simulink model "lab3sl"  (R2020b)
settings: Solver=VariableStepAuto  StartTime=0.0  StopTime=10.0  RelTol=1e-3
values from neighbouring files (symbols this model uses):
  a = t^3 * sin(2*t + pi)    [Laplace.m]    (also in lab3_config1 (1).m = 100)
  am = 1.71    [lab3_config1 (1).m]
  K = dcgain(num2,denum2)    [Lab2.m]    (also in Lab_4.m = 2.43; lab3_config1 (1).m = 22.985)
  K1 = 100    [lab3_config1 (1).m]
  Kg = 0.1    [lab3_config1 (1).m]
  Km = 2.083    [lab3_config1 (1).m]
  Kpot = 0.318    [lab3_config1 (1).m]
libraries: pid_lib x1
settings Model: Creator=mluser  LastModifiedBy=mluser

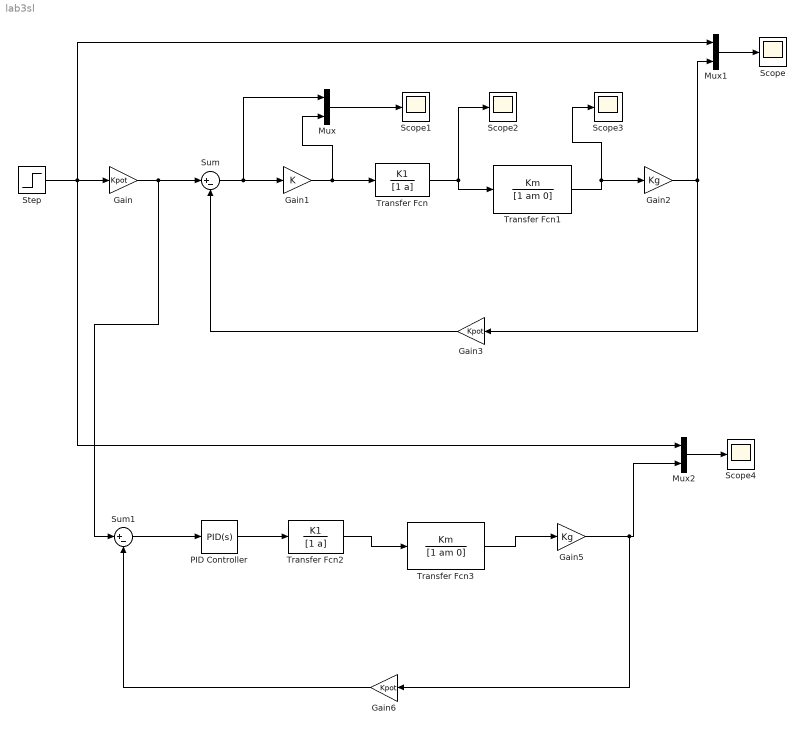
== system lab3sl ==
  Gain : Gain  Gain=Kpot
  Gain1 : Gain  Gain=K
  Gain2 : Gain  Gain=Kg
  Gain3 : Gain  Gain=Kpot
  Gain5 : Gain  Gain=Kg
  Gain6 : Gain  Gain=Kpot
  Mux : Mux  Inputs=2
  Mux1 : Mux  Inputs=2
  Mux2 : Mux  Inputs=2
  PID Controller : pid_lib/PID Controller  Controller=PID  Form=Parallel  TimeDomain=Continuous-time  UseExternalTs=off  SampleTime=-1  IntegratorMethod=Forward Euler  FilterMethod=Forward Euler  ControllerParametersSource=internal  P=1  I=1  D=0  UseFilter=on  N=100  TunerSelectOption=Transfer Function Based (PID Tuner App)  InitialConditionSource=internal  InitialConditionForIntegrator=0  InitialConditionForFilter=0  DifferentiatorICPrevScaledInput=0  ExternalReset=none  TrackingMode=off  Kt=1  LimitOutput=off  SatLimitsSource=internal  UpperSaturationLimit=inf  LowerSaturationLimit=-inf  LinearizeAsGain=on  AntiWindupMode=none  Kb=1  POutMin=[]  POutMax=[]  IOutMin=[]  IOutMax=[]  DOutMin=[]  DOutMax=[]  NOutMin=[]  NOutMax=[]  SumOutMin=[]  SumOutMax=[]  SaturationOutMin=[]  SaturationOutMax=[]  PParamMin=[]  PParamMax=[]  IParamMin=[]  IParamMax=[]  DParamMin=[]  DParamMax=[]  NParamMin=[]  NParamMax=[]  KbParamMin=[]  KbParamMax=[]  KtParamMin=[]  KtParamMax=[]  KbOutMin=[]  KbOutMax=[]  KtOutMin=[]  KtOutMax=[]  IntegratorOutMin=[]  IntegratorOutMax=[]  FilterOutMin=[]  FilterOutMax=[]  SumI1OutMin=[]  SumI1OutMax=[]  SumI2OutMin=[]  SumI2OutMax=[]  SumI3OutMin=[]  SumI3OutMax=[]  SumI4OutMin=[]  SumI4OutMax=[]  SumDOutMin=[]  SumDOutMax=[]  DifferentiatorOutMin=[]  DifferentiatorOutMax=[]  FilterDiffOutCoefMin=[]  FilterDiffOutCoefMax=[]  ReciprocalOutMin=[]  ReciprocalOutMax=[]  SumDenOutMin=[]  SumDenOutMax=[]  SumNumOutMin=[]  SumNumOutMax=[]  DivideOutMin=[]  DivideOutMax=[]  UdiffTsProdOutMin=[]  UdiffTsProdOutMax=[]  NTsProdOutMin=[]  NTsProdOutMax=[]  UintegralTsProdOutMin=[]  UintegralTsProdOutMax=[]  UngainTsProdOutMin=[]  UngainTsProdOutMax=[]  IntegratorContinuousStateAttributes=''  IntegratorStateMustResolveToSignalObject=off  IntegratorRTWStateStorageClass=Auto  FilterContinuousStateAttributes=''  FilterStateMustResolveToSignalObject=off  FilterRTWStateStorageClass=Auto  ParallelPVariant=InternalParameters  IdealPVariant=Disabled  IVariant=InternalParameters  DVariant=InternalParameters  IntegratorVariant=Continuous  SatVariant=Disabled  AWVariant=Passthrough  PCopyVariant=Disabled  TRVariant=Disabled  FdbkBlocksVariant=Forward  IdealPFdbkVariant=Disabled  SatFdbkVariant=Disabled  DerivativeFilterVariant=ContFilter  NVariant=InternalParameters  NCopyVariant=Disabled  FilterICVariant=InternalICsFilter  IntegratorICVariant=InternalICs  ExternalResetVariant=Disabled  TRSumVariant=Passthrough  SumFdbkVariant=Disabled  SumVariant=Sum_PID  TsampFilterVariant=InternalTs  TsampNgainVariant=Passthrough  TsampIntegralVariant=Passthrough  ExternalSaturationOutDataTypeStr=Inherit: Same as second input
  Scope{,1..4} (5 alike) : Scope
  Step : Step  After=0.5  SampleTime=0
  Sum : Sum  Inputs=|+-
  Sum1 : Sum  Inputs=|+-
  Transfer Fcn : TransferFcn  Numerator=K1  Denominator=[1 a]
  Transfer Fcn1 : TransferFcn  Numerator=Km  Denominator=[1 am 0]
  Transfer Fcn2 : TransferFcn  Numerator=K1  Denominator=[1 a]
  Transfer Fcn3 : TransferFcn  Numerator=Km  Denominator=[1 am 0]
  wires:
  Gain3/1 -> Sum/2
  Sum/1 -> Mux/1, Gain1/1
  Gain1/1 -> Mux/2, Transfer Fcn/1
  Transfer Fcn/1 -> Scope2/1, Transfer Fcn1/1
  Transfer Fcn1/1 -> Scope3/1, Gain2/1
  Mux/1 -> Scope1/1
  Mux1/1 -> Scope/1
  Gain2/1 -> Gain3/1, Mux1/2
  Gain6/1 -> Sum1/2
  Transfer Fcn2/1 -> Transfer Fcn3/1
  Gain/1 -> Sum1/1, Sum/1
  Sum1/1 -> PID Controller/1
  Transfer Fcn3/1 -> Gain5/1
  Mux2/1 -> Scope4/1
  Step/1 -> Mux2/1, Mux1/1, Gain/1
  Gain5/1 -> Gain6/1, Mux2/2
  PID Controller/1 -> Transfer Fcn2/1
